simulink model "simulazione_simulink_punto3"  (R2023a)
settings: Solver=VariableStepAuto  StartTime=0.0  StopTime=50  RelTol=1e-3
values from neighbouring files (symbols this model uses):
  A = [0,0,1,0 ; 0,0,0,1 ; -k/m1, k/m1, -c/m1, c/m1 ; k/m2, -k/m2, c/m2, -c/m2]    [Test.m]    (also in Test.mat = [0 0 -0.1 0.133333333333 0 0 0.1 -0.133333333333 1 0 -0.25 0)
  B = [0 ; 0 ; 1/m1 ; 0]    [Test.m]    (also in Test.mat = [0 0 0.0005 0])
  C = [1, 0, 0, 0]    [Test.m]    (also in Test.mat = [1 0 0 0])
  D = 0    [Test.m]
  g1 = 10    [Test.m]
  g2 = 0    [Test.m]
  g3 = 0    [Test.m]
  g4 = 0    [Test.m]
  L = 4    [Test.m]
  V = LV    [Test.m]
  x_0 = [0 ; 0 ; 0 ; 0]    [Test.m]
undefined symbols (not defined in the file or in its folder): gaussian
libraries: simulink x1
settings Model: Creator=Valeria  LastModifiedBy=Valeria

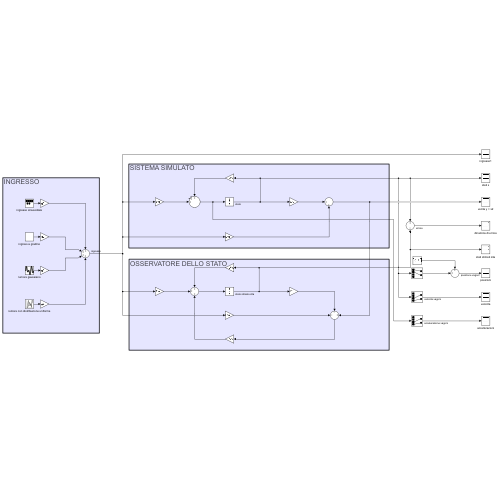
[thumbnail: Simulink's stored preview of the top-level diagram]
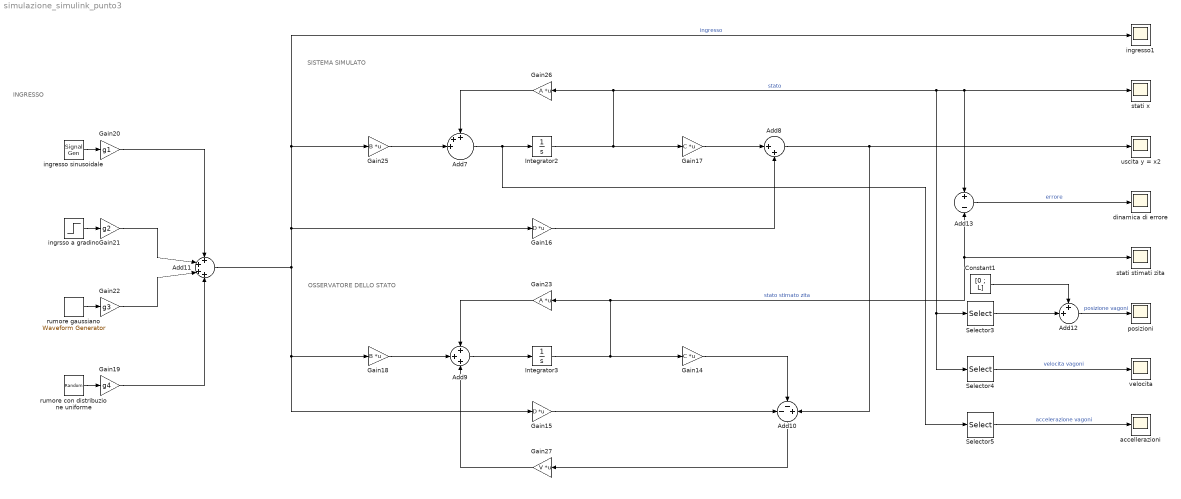
== system simulazione_simulink_punto3 ==
  note: SISTEMA SIMULATO
  note: OSSERVATORE DELLO STATO
  note: INGRESSO
  Add10 : Sum  Inputs=--+
  Add11 : Sum  Inputs=++++
  Add12 : Sum  Inputs=++|
  Add13 : Sum  Inputs=+-
  Add7 : Sum  Inputs=+++||
  Add8 : Sum  Inputs=|++
  Add9 : Sum  Inputs=+++
  Constant1 : Constant  Value=[0 ; L]
  Gain14 : Gain  Gain=C  Multiplication=Matrix(K*u)
  Gain15 : Gain  Gain=D  Multiplication=Matrix(K*u)
  Gain16 : Gain  Gain=D  Multiplication=Matrix(K*u)
  Gain17 : Gain  Gain=C  Multiplication=Matrix(K*u)
  Gain18 : Gain  Gain=B  Multiplication=Matrix(K*u)
  Gain19 : Gain  Gain=g4
  Gain20 : Gain  Gain=g1
  Gain21 : Gain  Gain=g2
  Gain22 : Gain  Gain=g3
  Gain23 : Gain  Gain=A  Multiplication=Matrix(K*u)
  Gain25 : Gain  Gain=B  Multiplication=Matrix(K*u)
  Gain26 : Gain  Gain=A  Multiplication=Matrix(K*u)
  Gain27 : Gain  Gain=V  Multiplication=Matrix(K*u)
  Integrator2 : Integrator  InitialCondition=x_0
  Integrator3 : Integrator  InitialCondition=[0 ; 0 ; 0 ; 0]
  Selector3 : Selector  InputPortWidth=4  IndexOptions=Index vector (dialog)  Indices=[1 2]  OutputSizes=1  RuntimeRangeChecks=on
  Selector4 : Selector  InputPortWidth=4  IndexOptions=Index vector (dialog)  Indices=[3 4]  OutputSizes=1  RuntimeRangeChecks=on
  Selector5 : Selector  InputPortWidth=4  IndexOptions=Index vector (dialog)  Indices=[3 4]  OutputSizes=1  RuntimeRangeChecks=on
  accellerazioni : Scope
  dinamica di errore : Scope
  ingresso sinusoidale : SignalGenerator
  ingresso1 : Scope
  ingrsso a gradino : Step  Time=0  SampleTime=0  ZeroCross=off
  posizioni : Scope
  rumore con distribuzione uniforme : UniformRandomNumber  SampleTime=0.1
  rumore gaussiano : simulink/Sources/Waveform Generator  OutMin=[]  OutMax=[]  OutDataTypeStr=double  SelectedSignal=1  Signals=gaussian()  BlockNames=MultiportSwitch_746ec0809bf24cb  SampleTime=0.1
  stati stimati zita : Scope
  stati x : Scope
  uscita y = x2 : Scope
  velocita : Scope
  wires:
  Selector3/1 -> Add12/2
  Add12/1 -> posizioni/1  "posizione vagoni"
  Gain19/1 -> Add11/4
  ingrsso a gradino/1 -> Gain21/1
  Add11/1 -> Gain15/1, Gain18/1, Gain16/1, ingresso1/1, Gain25/1  "ingresso"
  Add7/1 -> Selector5/1, Integrator2/1
  Gain23/1 -> Add9/1
  Add10/1 -> Gain27/1
  Gain27/1 -> Add9/3
  Gain25/1 -> Add7/3
  Integrator3/1 -> Gain23/1, Add13/2, stati stimati zita/1, Gain14/1  "stato stimato zita"
  Add9/1 -> Integrator3/1
  Gain26/1 -> Add7/1
  Gain16/1 -> Add8/2
  rumore gaussiano/1 -> Gain22/1
  Gain21/1 -> Add11/2
  ingresso sinusoidale/1 -> Gain20/1
  Gain14/1 -> Add10/2
  Add8/1 -> Add10/3, uscita y = x2/1
  Integrator2/1 -> Gain17/1, Selector3/1, Selector4/1, stati x/1, Add13/1, Gain26/1  "stato"
  Gain20/1 -> Add11/1
  Gain18/1 -> Add9/2
  rumore con distribuzione uniforme/1 -> Gain19/1
  Gain15/1 -> Add10/1
  Selector4/1 -> velocita/1  "velocita vagoni"
  Gain17/1 -> Add8/1
  Add13/1 -> dinamica di errore/1  "errore"
  Constant1/1 -> Add12/1
  Gain22/1 -> Add11/3
  Selector5/1 -> accellerazioni/1  "accelerazione vagoni"
